simulink model "rs_bicycle_old"  (R2019b)
settings: Solver=FixedStepAuto  StartTime=0.0  StopTime=200  FixedStep=0.1  RelTol=1e-3
undefined symbols (not defined in the file): duration, env_forest, env_mu_s_dry, env_mu_s_wet, env_route_length, env_t_rain_start, env_traffic_durations, env_traffic_pos, env_traffic_times, g, init_position, init_velocity, limit_velocity
libraries: dspstat3 x6, simulink x1
settings Model: Creator=ggarrett  LastModifiedBy=ggarrett
settings DataIOCC: ExternalInput=[x]  SaveFormat=Array  SaveTime=off  OutputSaveName=f
settings OptimizationCC: OptimizeBlockIOStorage=off  BufferReuse=off  GlobalBufferReuse=off  ExpressionFolding=off  LocalBlockOutputs=off  OptimizeDataStoreBuffers=off  BusAssignmentInplaceUpdate=off
settings DebuggingCC: SFUnexpectedBacktrackingDiag=warning  SFNoUnconditionalDefaultTransitionDiag=warning
settings HardwareCC: ProdBitPerLong=64  ProdHWDeviceType=Intel->x86-64 (Linux 64)  TargetBitPerLong=64  TargetBitPerPointer=64  TargetBitPerSizeT=64  TargetBitPerPtrDiffT=64  TargetLongLongMode=on  TargetIntDivRoundTo=Zero  TargetEndianess=LittleEndian  TargetWordSize=64  TargetHWDeviceType=MATLAB Host  ProdEqTarget=off
settings RTWCC: Description=Rapid Simulation Target  SystemTargetFile=rsim.tlc  TemplateMakefile=rsim_default_tmf  GenerateReport=on  BuildConfiguration=Debug  LaunchReport=on
settings CodeAppCC: ForceParamTrailComments=on  MATLABSourceComments=on  EnableCustomComments=on
settings RSimTargetCC: TargetLangStandard=C99 (ISO)  GeneratePreprocessorConditionals=Use local settings  PreserveStateflowLocalDataDimensions=off

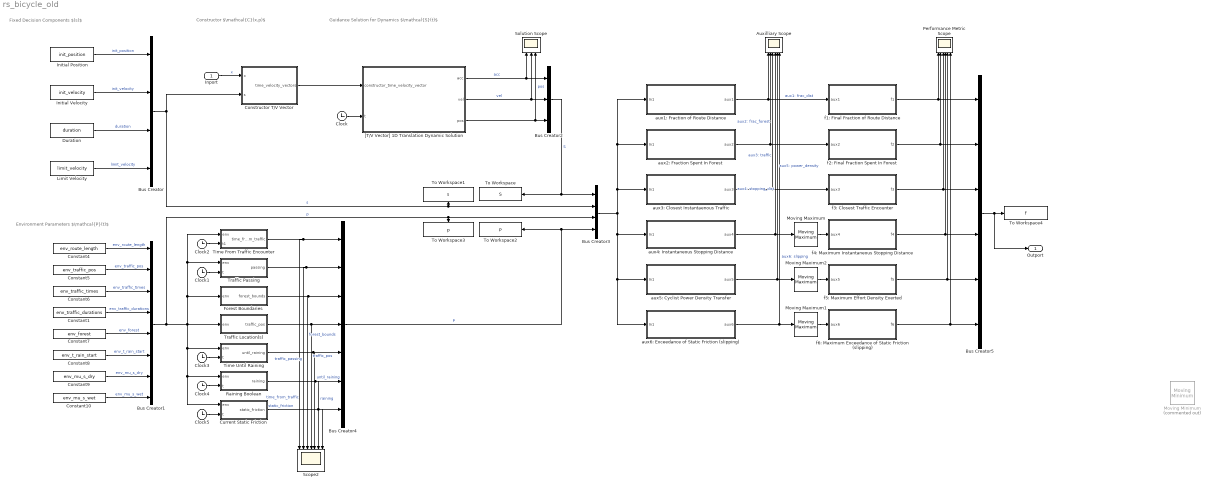
== system rs_bicycle_old ==
  note: Guidance Solution for Dynamics $\mathcal{S}(t)$
  note: Fixed Decision Components $(s)$
  note: Environment Parameters $\mathcal{P}(t)$
  note: Constructor $\mathcal{C}(x,p)$
  Inport : Inport  OutDataTypeStr=double  PortDimensions=6
  Auxilliary Scope : Scope  NumInputPorts=6
  Bus Creator : BusCreator  Inputs=4
  Bus Creator1 : BusCreator  Inputs=8
  Bus Creator2 : BusCreator  Inputs=3
  Bus Creator3 : BusCreator  Inputs=4
  Bus Creator4 : BusCreator  Inputs=7
  Bus Creator5 : BusCreator  Inputs=6
  Clock{,1..5} (6 alike) : Clock
  Constant1 : Constant  Value=env_traffic_durations
  Constant10 : Constant  Value=env_mu_s_wet
  Constant4 : Constant  Value=env_route_length
  Constant5 : Constant  Value=env_traffic_pos
  Constant6 : Constant  Value=env_traffic_times
  Constant7 : Constant  Value=env_forest
  Constant8 : Constant  Value=env_t_rain_start
  Constant9 : Constant  Value=env_mu_s_dry
  Constructor T/V Vector : Subsystem
  Current Static Friction : Subsystem
  Duration : Constant  Value=duration
  Forest Boundaries : Subsystem
  Initial Position : Constant  Value=init_position
  Initial Velocity : Constant  Value=init_velocity
  Limit Velocity : Constant  Value=limit_velocity
  Moving Maximum : dspstat3/Moving Maximum  SpecifyWindowLength=on  WindowLength=duration  SimulateUsing=Code generation
      settings: SourceProductName=DSP System Toolbox  SourceProductBaseCode=DS
  Moving Maximum1 : dspstat3/Moving Maximum  SpecifyWindowLength=on  WindowLength=duration  SimulateUsing=Code generation
      settings: SourceProductName=DSP System Toolbox  SourceProductBaseCode=DS
  Moving Maximum2 : dspstat3/Moving Maximum  SpecifyWindowLength=on  WindowLength=duration  SimulateUsing=Code generation
      settings: SourceProductName=DSP System Toolbox  SourceProductBaseCode=DS
  Moving Minimum : dspstat3/Moving Minimum  Commented=on  SpecifyWindowLength=on  WindowLength=4  SimulateUsing=Code generation
      settings: SourceProductName=DSP System Toolbox  SourceProductBaseCode=DS
  Performance Metric Scope : Scope  NumInputPorts=6
  Raining Boolean : Subsystem
  Scope2 : Scope  NumInputPorts=7
  Solution Scope : Scope  NumInputPorts=3
  Time From Traffic Encounter : Subsystem
  Time Until Raining : Subsystem
  To Workspace : ToWorkspace  VariableName=S  SaveFormat=Timeseries  SampleTime=-1
  To Workspace1 : ToWorkspace  VariableName=s  SaveFormat=Timeseries  SampleTime=-1
  To Workspace2 : ToWorkspace  VariableName=P  SaveFormat=Timeseries  SampleTime=-1
  To Workspace3 : ToWorkspace  VariableName=p  SaveFormat=Timeseries  SampleTime=-1
  To Workspace4 : ToWorkspace  VariableName=f  SaveFormat=Timeseries  SampleTime=-1
  Traffic Location(s) : Subsystem
  Traffic Passing : Subsystem
  "[T/V Vector] 1D Translation Dynamic Solution" : Subsystem
  aux1: Fraction of Route Distance : Subsystem
  aux2: Fraction Spent In Forest : Subsystem
  aux3: Closest Instantaenous Traffic : Subsystem
  aux4: Instantaneous Stopping Distance : Subsystem
  aux5: Cyclist Power Density Transfer : Subsystem
  aux6: Exceedance of Static Friction (slipping) : Subsystem
  f1: Final Fraction of Route Distance : Subsystem
  f2: Final Fraction Spent In Forest : Subsystem
  "f3: Closest Traffic Encounter " : Subsystem
  f4: Maximum Instantaneous Stopping Distance : Subsystem
  f5: Maximum Effort Density Exerted : Subsystem
  f6: Maximum Exceedance of Static Friction (slipping) : Subsystem
  Outport : Outport
  wires:
  Initial Position/1 -> Bus Creator/1  "init_position"
  Initial Velocity/1 -> Bus Creator/2  "init_velocity"
  Constant4/1 -> Bus Creator1/1  "env_route_length"
  Constant5/1 -> Bus Creator1/2  "env_traffic_pos"
  Constant6/1 -> Bus Creator1/3  "env_traffic_times"
  Constant7/1 -> Bus Creator1/5  "env_forest"
  Constant9/1 -> Bus Creator1/7  "env_mu_s_dry"
  Constant8/1 -> Bus Creator1/6  "env_t_rain_start"
  Constant10/1 -> Bus Creator1/8  "env_mu_s_wet"
  Bus Creator1/1 -> Time From Traffic Encounter/1(env), Traffic Passing/1(env), Forest Boundaries/1(env), Traffic Location(s)/1(env), Current Static Friction/1(env), Raining Boolean/1(env), Time Until Raining/1(env), To Workspace3/1, Bus Creator3/3  "p"
  Duration/1 -> Bus Creator/3  "duration"
  Limit Velocity/1 -> Bus Creator/4  "limit_velocity"
  Inport/1 -> Constructor T/V Vector/1(x)  "x"
  Bus Creator/1 -> Constructor T/V Vector/2(s), To Workspace1/1, Bus Creator3/2  "s"
  Clock/1 -> "[T/V Vector] 1D Translation Dynamic Solution"/2(t)
  "[T/V Vector] 1D Translation Dynamic Solution"/2(vel) -> Bus Creator2/2, Solution Scope/2  "vel"
  "[T/V Vector] 1D Translation Dynamic Solution"/3(pos) -> Bus Creator2/3, Solution Scope/3  "pos"
  Clock1/1 -> Traffic Passing/2(t)
  Clock2/1 -> Time From Traffic Encounter/2(t1)
  Clock3/1 -> Time Until Raining/2(t)
  Clock4/1 -> Raining Boolean/2(t)
  Clock5/1 -> Current Static Friction/2(t)
  Constructor T/V Vector/1(time_velocity_vectors) -> "[T/V Vector] 1D Translation Dynamic Solution"/1(constructor_time_velocity_vector)
  Time From Traffic Encounter/1(time_from_traffic) -> Scope2/1, Bus Creator4/1  "time_from_traffic"
  Traffic Passing/1(passing) -> Scope2/2, Bus Creator4/2  "traffic_passing"
  Forest Boundaries/1(forest_bounds) -> Scope2/3, Bus Creator4/3  "forest_bounds"
  Traffic Location(s)/1(traffic_pos) -> Scope2/4, Bus Creator4/4  "traffic_pos"
  Time Until Raining/1(until_raining) -> Scope2/5, Bus Creator4/5  "until_raining"
  Raining Boolean/1(raining) -> Scope2/6, Bus Creator4/6  "raining"
  Current Static Friction/1(static_friction) -> Scope2/7, Bus Creator4/7  "static_friction"
  Bus Creator4/1 -> To Workspace2/1, Bus Creator3/4  "P"
  "[T/V Vector] 1D Translation Dynamic Solution"/1(acc) -> Bus Creator2/1, Solution Scope/1  "acc"
  Bus Creator2/1 -> Bus Creator3/1, To Workspace/1  "S"
  Bus Creator3/1 -> aux1: Fraction of Route Distance/1(In1), aux2: Fraction Spent In Forest/1(In1), aux3: Closest Instantaenous Traffic/1(In1), aux6: Exceedance of Static Friction (slipping)/1(In1), aux5: Cyclist Power Density Transfer/1(In1), aux4: Instantaneous Stopping Distance/1(In1)
  Constant1/1 -> Bus Creator1/4  "env_traffic_durations"
  aux1: Fraction of Route Distance/1(aux1) -> Auxilliary Scope/1, f1: Final Fraction of Route Distance/1(aux1)  "aux1: frac_dist"
  aux2: Fraction Spent In Forest/1(aux2) -> f2: Final Fraction Spent In Forest/1(aux2), Auxilliary Scope/2  "aux2: frac_forest"
  aux3: Closest Instantaenous Traffic/1(aux3) -> "f3: Closest Traffic Encounter "/1(aux3), Auxilliary Scope/3  "aux3: traffic"
  aux4: Instantaneous Stopping Distance/1(aux4) -> Moving Maximum/1, Auxilliary Scope/4  "aux4: stopping_dist"
  aux5: Cyclist Power Density Transfer/1(aux5) -> Moving Maximum2/1, Auxilliary Scope/5  "aux5: power_density"
  aux6: Exceedance of Static Friction (slipping)/1(aux6) -> Moving Maximum1/1, Auxilliary Scope/6  "aux6: slipping"
  Moving Maximum/1 -> f4: Maximum Instantaneous Stopping Distance/1(aux4)
  Moving Maximum1/1 -> f6: Maximum Exceedance of Static Friction (slipping)/1(aux6)
  f6: Maximum Exceedance of Static Friction (slipping)/1(f6) -> Bus Creator5/6, Performance Metric Scope/6
  f1: Final Fraction of Route Distance/1(f1) -> Performance Metric Scope/1, Bus Creator5/1
  f2: Final Fraction Spent In Forest/1(f2) -> Performance Metric Scope/2, Bus Creator5/2
  "f3: Closest Traffic Encounter "/1(f3) -> Performance Metric Scope/3, Bus Creator5/3
  f4: Maximum Instantaneous Stopping Distance/1(f4) -> Performance Metric Scope/4, Bus Creator5/4
  f5: Maximum Effort Density Exerted/1(f5) -> Performance Metric Scope/5, Bus Creator5/5
  Bus Creator5/1 -> Outport/1, To Workspace4/1
  Moving Maximum2/1 -> f5: Maximum Effort Density Exerted/1(aux5)

== system rs_bicycle_old/Constructor T//V Vector ==
  x : Inport
  s : Inport  Port=2
  Bus Creator : BusCreator  Inputs=2
  Velocity and Time Vectors : MATLAB Function  TreatAsAtomicUnit=on
  time_velocity_vectors : Outport
  wires:
  s/1 -> Velocity and Time Vectors/2(s)
  x/1 -> Velocity and Time Vectors/1(x)
  Velocity and Time Vectors/2(velocities) -> Bus Creator/2  "velocities"
  Velocity and Time Vectors/1(times) -> Bus Creator/1  "times"
  Bus Creator/1 -> time_velocity_vectors/1  "time_velocity_vectors"

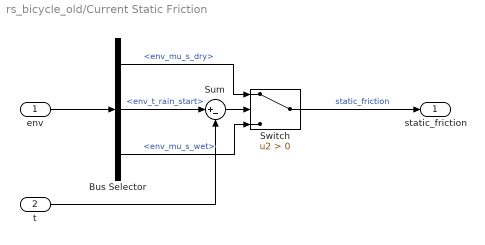
== system rs_bicycle_old/Current Static Friction ==
  env : Inport
  t : Inport  Port=2
  Bus Selector : BusSelector  OutputSignals=env_mu_s_dry,env_t_rain_start,env_mu_s_wet
  Sum : Sum  Inputs=|+-
  Switch : Switch  Criteria=u2 > Threshold
  static_friction : Outport
  wires:
  Bus Selector/2 -> Sum/1  "<env_t_rain_start>"
  t/1 -> Sum/2
  Bus Selector/1 -> Switch/1  "<env_mu_s_dry>"
  Sum/1 -> Switch/2
  env/1 -> Bus Selector/1
  Bus Selector/3 -> Switch/3  "<env_mu_s_wet>"
  Switch/1 -> static_friction/1  "static_friction"

== system rs_bicycle_old/Forest Boundaries ==
  env : Inport
  Bus Selector : BusSelector  OutputSignals=env_forest,env_route_length
  Product : Product
  forest_bounds : Outport
  wires:
  Bus Selector/1 -> Product/1  "<env_forest>"
  Bus Selector/2 -> Product/2  "<env_route_length>"
  Product/1 -> forest_bounds/1
  env/1 -> Bus Selector/1

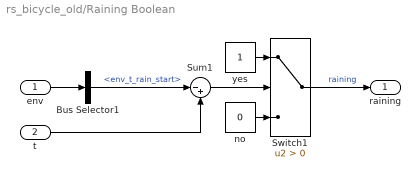
== system rs_bicycle_old/Raining Boolean ==
  env : Inport
  t : Inport  Port=2
  Bus Selector1 : BusSelector  OutputSignals=env_t_rain_start
  Sum1 : Sum  Inputs=|-+
  Switch1 : Switch  Criteria=u2 > Threshold
  no : Constant  Value=0
  yes : Constant
  raining : Outport
  wires:
  yes/1 -> Switch1/1
  Bus Selector1/1 -> Sum1/1  "<env_t_rain_start>"
  no/1 -> Switch1/3
  Switch1/1 -> raining/1  "raining"
  env/1 -> Bus Selector1/1
  Sum1/1 -> Switch1/2
  t/1 -> Sum1/2

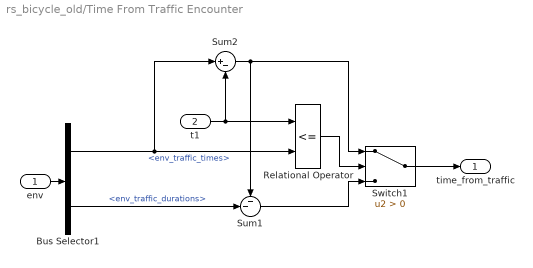
== system rs_bicycle_old/Time From Traffic Encounter ==
  env : Inport
  t1 : Inport  Port=2
  Bus Selector1 : BusSelector  OutputSignals=env_traffic_times,env_traffic_durations
  Relational Operator : RelationalOperator  Operator=<=  OutDataTypeStr=boolean  RndMeth=Simplest
  Sum1 : Sum  Inputs=--|
  Sum2 : Sum  Inputs=|+-
  Switch1 : Switch  Criteria=u2 > Threshold
  time_from_traffic : Outport
  wires:
  Bus Selector1/2 -> Sum1/2  "<env_traffic_durations>"
  Bus Selector1/1 -> Relational Operator/2, Sum2/1  "<env_traffic_times>"
  Switch1/1 -> time_from_traffic/1
  env/1 -> Bus Selector1/1
  Sum1/1 -> Switch1/3
  Sum2/1 -> Sum1/1, Switch1/1
  Relational Operator/1 -> Switch1/2
  t1/1 -> Relational Operator/1, Sum2/2

== system rs_bicycle_old/Time Until Raining ==
  env : Inport
  t : Inport  Port=2
  Bus Selector1 : BusSelector  OutputSignals=env_t_rain_start
  Sum1 : Sum  Inputs=|+-
  until_raining : Outport
  wires:
  Bus Selector1/1 -> Sum1/1  "<env_t_rain_start>"
  env/1 -> Bus Selector1/1
  t/1 -> Sum1/2
  Sum1/1 -> until_raining/1

== system rs_bicycle_old/Traffic Location(s) ==
  env : Inport
  Bus Selector : BusSelector  OutputSignals=env_traffic_pos,env_route_length
  Product : Product
  traffic_pos : Outport
  wires:
  Bus Selector/1 -> Product/1  "<env_traffic_pos>"
  Bus Selector/2 -> Product/2  "<env_route_length>"
  Product/1 -> traffic_pos/1
  env/1 -> Bus Selector/1

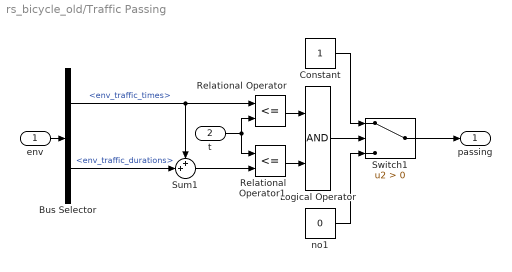
== system rs_bicycle_old/Traffic Passing ==
  env : Inport
  t : Inport  Port=2
  Bus Selector : BusSelector  OutputSignals=env_traffic_times,env_traffic_durations
  Constant : Constant
  Logical Operator : Logic  AllPortsSameDT=off  OutDataTypeStr=boolean
  Relational Operator : RelationalOperator  Operator=<=  OutDataTypeStr=boolean  RndMeth=Simplest
  Relational Operator1 : RelationalOperator  Operator=<=  OutDataTypeStr=boolean  RndMeth=Simplest
  Sum1 : Sum  Inputs=++|
  Switch1 : Switch  Criteria=u2 > Threshold
  no1 : Constant  Value=0
  passing : Outport
  wires:
  env/1 -> Bus Selector/1
  Logical Operator/1 -> Switch1/2
  Relational Operator1/1 -> Logical Operator/2
  t/1 -> Relational Operator/2, Relational Operator1/1
  no1/1 -> Switch1/3
  Relational Operator/1 -> Logical Operator/1
  Switch1/1 -> passing/1
  Constant/1 -> Switch1/1
  Sum1/1 -> Relational Operator1/2
  Bus Selector/1 -> Sum1/1, Relational Operator/1  "<env_traffic_times>"
  Bus Selector/2 -> Sum1/2  "<env_traffic_durations>"

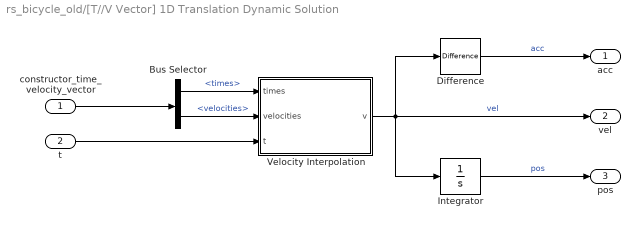
== system rs_bicycle_old/[T//V Vector] 1D Translation Dynamic Solution ==
  constructor_time_velocity_vector : Inport
  t : Inport  Port=2
  Bus Selector : BusSelector  OutputSignals=times,velocities
  Difference : simulink/Discrete/Difference  ICPrevInput=0.0  OutMin=[]  OutMax=[]  OutDataType=fixdt(1, 16)  OutScaling=2^-10  RndMeth=Round  DoSatur=off
  Integrator : Integrator  InitialCondition=init_position
  Velocity Interpolation : MATLAB Function  TreatAsAtomicUnit=on
  acc : Outport
  vel : Outport  Port=2
  pos : Outport  Port=3
  wires:
  Bus Selector/2 -> Velocity Interpolation/2(velocities)  "<velocities>"
  Velocity Interpolation/1(v) -> vel/1, Integrator/1, Difference/1  "vel"
  Difference/1 -> acc/1  "acc"
  t/1 -> Velocity Interpolation/3(t)
  Integrator/1 -> pos/1  "pos"
  Bus Selector/1 -> Velocity Interpolation/1(times)  "<times>"
  constructor_time_velocity_vector/1 -> Bus Selector/1

== system rs_bicycle_old/aux1: Fraction of Route Distance ==
  In1 : Inport
  Bus Selector : BusSelector  OutputSignals=S.pos,p.env_route_length
  Divide : Product  Inputs=*/
  Moving Maximum : dspstat3/Moving Maximum  SpecifyWindowLength=on  WindowLength=4  SimulateUsing=Code generation
      settings: SourceProductName=DSP System Toolbox  SourceProductBaseCode=DS
  aux1 : Outport
  wires:
  Divide/1 -> aux1/1  "frac_dist"
  In1/1 -> Bus Selector/1
  Bus Selector/2 -> Divide/2  "<env_route_length>"
  Bus Selector/1 -> Moving Maximum/1  "<pos>"
  Moving Maximum/1 -> Divide/1

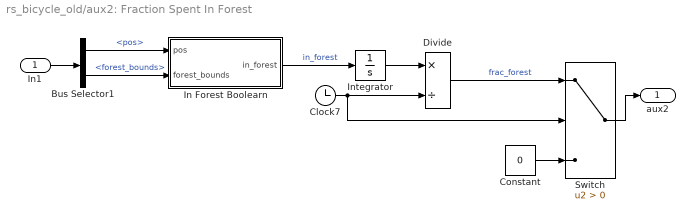
== system rs_bicycle_old/aux2: Fraction Spent In Forest ==
  In1 : Inport
  Bus Selector1 : BusSelector  OutputSignals=S.pos,P.forest_bounds
  Clock7 : Clock
  Constant : Constant  Value=0
  Divide : Product  Inputs=*/
  In Forest Boolearn : Subsystem
  Integrator : Integrator
  Switch : Switch  Criteria=u2 > Threshold
  aux2 : Outport
  wires:
  Integrator/1 -> Divide/1
  Bus Selector1/1 -> In Forest Boolearn/1("pos ")  "<pos>"
  In1/1 -> Bus Selector1/1
  Clock7/1 -> Switch/2, Divide/2
  In Forest Boolearn/1("in_forest ") -> Integrator/1  "in_forest"
  Bus Selector1/2 -> In Forest Boolearn/2(forest_bounds)  "<forest_bounds>"
  Divide/1 -> Switch/1  "frac_forest"
  Switch/1 -> aux2/1
  Constant/1 -> Switch/3

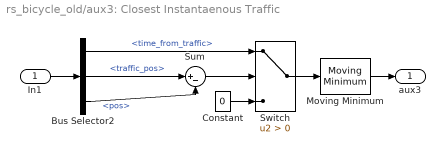
== system rs_bicycle_old/aux3: Closest Instantaenous Traffic ==
  In1 : Inport
  Bus Selector2 : BusSelector  OutputSignals=P.time_from_traffic,P.traffic_pos,S.pos
  Constant : Constant  Value=0
  Moving Minimum : dspstat3/Moving Minimum  SpecifyWindowLength=on  WindowLength=500  SimulateUsing=Code generation
      settings: SourceProductName=DSP System Toolbox  SourceProductBaseCode=DS
  Sum : Sum  Inputs=|+-
  Switch : Switch  Criteria=u2 > Threshold
  aux3 : Outport
  wires:
  Switch/1 -> Moving Minimum/1
  Bus Selector2/1 -> Switch/1  "<time_from_traffic>"
  In1/1 -> Bus Selector2/1
  Moving Minimum/1 -> aux3/1
  Sum/1 -> Switch/2
  Constant/1 -> Switch/3
  Bus Selector2/3 -> Sum/2  "<pos>"
  Bus Selector2/2 -> Sum/1  "<traffic_pos>"

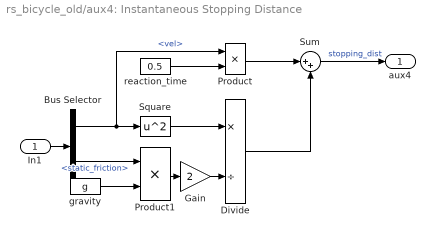
== system rs_bicycle_old/aux4: Instantaneous Stopping Distance ==
  In1 : Inport
  Bus Selector : BusSelector  OutputSignals=S.vel,P.static_friction
  Divide : Product  Inputs=*/
  Gain : Gain  Gain=2
  Product : Product
  Product1 : Product
  Square : Math  Operator=square  SignedPower=off  SaturateOnIntegerOverflow=on
  Sum : Sum  Inputs=|++
  gravity : Constant  Value=g
  reaction_time : Constant  Value=0.5
  aux4 : Outport
  wires:
  Bus Selector/2 -> Product1/1  "<static_friction>"
  Sum/1 -> aux4/1  "stopping_dist"
  Product/1 -> Sum/1
  Divide/1 -> Sum/2
  Square/1 -> Divide/1
  In1/1 -> Bus Selector/1
  Bus Selector/1 -> Product/1, Square/1  "<vel>"
  gravity/1 -> Product1/2
  Gain/1 -> Divide/2
  Product1/1 -> Gain/1
  reaction_time/1 -> Product/2

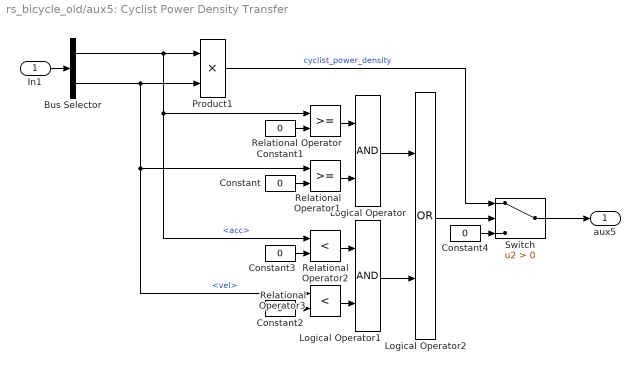
== system rs_bicycle_old/aux5: Cyclist Power Density Transfer ==
  In1 : Inport
  Bus Selector : BusSelector  OutputSignals=S.acc,S.vel
  Constant{,1..4} (5 alike) : Constant  Value=0
  Logical Operator : Logic  AllPortsSameDT=off  OutDataTypeStr=boolean
  Logical Operator1 : Logic  AllPortsSameDT=off  OutDataTypeStr=boolean
  Logical Operator2 : Logic  Operator=OR  AllPortsSameDT=off  OutDataTypeStr=boolean
  Product1 : Product
  Relational Operator : RelationalOperator  OutDataTypeStr=boolean  RndMeth=Simplest
  Relational Operator1 : RelationalOperator  OutDataTypeStr=boolean  RndMeth=Simplest
  Relational Operator2 : RelationalOperator  Operator=<  OutDataTypeStr=boolean  RndMeth=Simplest
  Relational Operator3 : RelationalOperator  Operator=<  OutDataTypeStr=boolean  RndMeth=Simplest
  Switch : Switch  Criteria=u2 > Threshold
  aux5 : Outport
  wires:
  Bus Selector/2 -> Relational Operator3/1, Relational Operator1/1, Product1/2  "<vel>"
  Product1/1 -> Switch/1  "cyclist_power_density"
  Bus Selector/1 -> Relational Operator2/1, Relational Operator/1, Product1/1  "<acc>"
  In1/1 -> Bus Selector/1
  Relational Operator/1 -> Logical Operator/1
  Relational Operator1/1 -> Logical Operator/2
  Constant/1 -> Relational Operator1/2
  Constant1/1 -> Relational Operator/2
  Constant2/1 -> Relational Operator3/2
  Relational Operator3/1 -> Logical Operator1/2
  Constant3/1 -> Relational Operator2/2
  Relational Operator2/1 -> Logical Operator1/1
  Logical Operator1/1 -> Logical Operator2/2
  Logical Operator/1 -> Logical Operator2/1
  Logical Operator2/1 -> Switch/2
  Switch/1 -> aux5/1
  Constant4/1 -> Switch/3

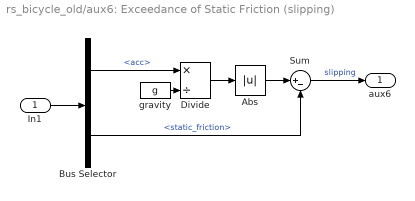
== system rs_bicycle_old/aux6: Exceedance of Static Friction (slipping) ==
  In1 : Inport
  Abs : Abs
  Bus Selector : BusSelector  OutputSignals=S.acc,P.static_friction
  Divide : Product  Inputs=*/
  Sum : Sum  Inputs=|+-
  gravity : Constant  Value=g
  aux6 : Outport
  wires:
  Bus Selector/1 -> Divide/1  "<acc>"
  Bus Selector/2 -> Sum/2  "<static_friction>"
  In1/1 -> Bus Selector/1
  Sum/1 -> aux6/1  "slipping"
  Divide/1 -> Abs/1
  gravity/1 -> Divide/2
  Abs/1 -> Sum/1

== system rs_bicycle_old/f1: Final Fraction of Route Distance ==
  aux1 : Inport
  Clock6 : Clock
  Memory : Memory
  Switch : Switch  Threshold=duration
  f1 : Outport
  wires:
  Clock6/1 -> Switch/2
  Memory/1 -> Switch/3
  Switch/1 -> f1/1, Memory/1
  aux1/1 -> Switch/1

== system rs_bicycle_old/f2: Final Fraction Spent In Forest ==
  aux2 : Inport
  Clock6 : Clock
  Memory : Memory
  Switch : Switch  Threshold=duration
  f2 : Outport
  wires:
  Clock6/1 -> Switch/2
  Memory/1 -> Switch/3
  Switch/1 -> f2/1, Memory/1
  aux2/1 -> Switch/1

== system rs_bicycle_old/f3: Closest Traffic Encounter  ==
  aux3 : Inport
  Clock6 : Clock
  Memory : Memory
  Switch : Switch  Threshold=duration
  f3 : Outport
  wires:
  Clock6/1 -> Switch/2
  Memory/1 -> Switch/3
  Switch/1 -> f3/1, Memory/1
  aux3/1 -> Switch/1

== system rs_bicycle_old/f4: Maximum Instantaneous Stopping Distance ==
  aux4 : Inport
  Clock6 : Clock
  Memory : Memory
  Switch : Switch  Threshold=duration
  f4 : Outport
  wires:
  Clock6/1 -> Switch/2
  Memory/1 -> Switch/3
  Switch/1 -> f4/1, Memory/1
  aux4/1 -> Switch/1

== system rs_bicycle_old/f5: Maximum Effort Density Exerted ==
  aux5 : Inport
  Clock6 : Clock
  Memory : Memory
  Switch : Switch  Threshold=duration
  f5 : Outport
  wires:
  Clock6/1 -> Switch/2
  Memory/1 -> Switch/3
  Switch/1 -> f5/1, Memory/1
  aux5/1 -> Switch/1

== system rs_bicycle_old/f6: Maximum Exceedance of Static Friction (slipping) ==
  aux6 : Inport
  Clock6 : Clock
  Memory : Memory
  Switch : Switch  Threshold=duration
  f6 : Outport
  wires:
  Clock6/1 -> Switch/2
  Memory/1 -> Switch/3
  Switch/1 -> f6/1, Memory/1
  aux6/1 -> Switch/1

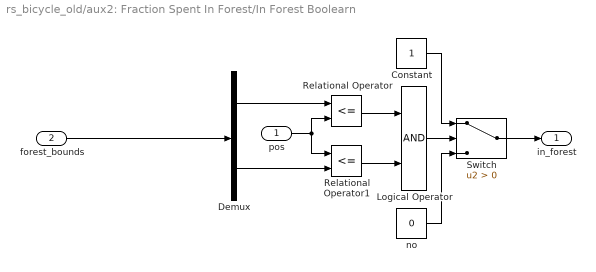
== system rs_bicycle_old/aux2: Fraction Spent In Forest/In Forest Boolearn ==
  "pos " : Inport
  forest_bounds : Inport  Port=2
  Constant : Constant
  Demux : Demux  Outputs=2
  Logical Operator : Logic  AllPortsSameDT=off  OutDataTypeStr=boolean
  Relational Operator : RelationalOperator  Operator=<=  OutDataTypeStr=boolean  RndMeth=Simplest
  Relational Operator1 : RelationalOperator  Operator=<=  OutDataTypeStr=boolean  RndMeth=Simplest
  Switch : Switch  Criteria=u2 > Threshold
  no : Constant  Value=0
  "in_forest " : Outport
  wires:
  Switch/1 -> "in_forest "/1
  Relational Operator/1 -> Logical Operator/1
  Relational Operator1/1 -> Logical Operator/2
  forest_bounds/1 -> Demux/1
  Logical Operator/1 -> Switch/2
  "pos "/1 -> Relational Operator/2, Relational Operator1/1
  Demux/1 -> Relational Operator/1
  Demux/2 -> Relational Operator1/2
  Constant/1 -> Switch/1
  no/1 -> Switch/3

== matlab function rs_bicycle_old/[T//V Vector] 1D Translation Dynamic Solution/Velocity Interpolation ==
  data: times input; v output; velocities input; t input
function v = fcn(times, velocities, t)

v = interp1(times, velocities, t);

== matlab function rs_bicycle_old/Constructor T//V Vector/Velocity and Time Vectors ==
  data: x input; s input; times output; velocities output
function [times, velocities]= constructor(x, s) %#codegen

initial_velocity = s(2);
duration = s(3);
limit_v = s(4);

n_x = max(size(x));
n_v = n_x/2;

times_ = x(n_v+1:end) + 0.01;
times = cumsum([0; times_]);
times = times / max(times);
times = times * duration;
% 
velocities_ = x(1:n_v) * limit_v;
velocities = [initial_velocity; velocities_];
%
